simulink model "matlab_smith_opc_opre"  (R2018b)
settings: Solver=VariableStepAuto  StartTime=0.0  StopTime=40  RelTol=1e-3
undefined symbols (not defined in the file or in its folder): AI1, AO1, Dev1
libraries: opclib x3, simulink x1
settings Model: Creator=erange  LastModifiedBy=erange

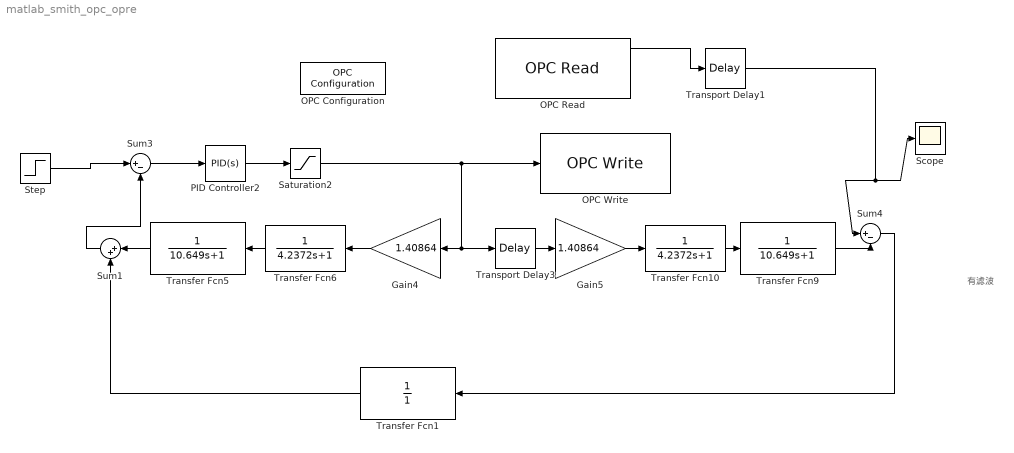
== system matlab_smith_opc_opre ==
  note: 有滤波
  Gain4 : Gain  Gain=1.40864
  Gain5 : Gain  Gain=1.40864
  OPC Configuration : opclib/OPC Configuration  opcServers=localhost/NI USB-6008.Server/10, localhost/Tank2.Server/10  errMissingItems=Error  errReadWrite=Warn  errShutdown=Error  errRTViolation=Warn  rtEnable=on  speedup=1  showLatency=off  beingUsed=on
      settings: SourceProductName=OPC Toolbox  SourceProductBaseCode=OT
  OPC Read : opclib/OPC Read  serverHost=localhost  serverID=NI USB-6008.Server  itemIDs=Dev1/AI1  readMode=Synchronous (cache)  dataType=double  updateRate=0.01  showQual=on  showTS=on  tsMode=Seconds since start
      settings: SourceProductName=OPC Toolbox  SourceProductBaseCode=OT
  OPC Write : opclib/OPC Write  serverHost=localhost  serverID=NI USB-6008.Server  itemIDs=Dev1/AO1  writeMode=Synchronous  updateRate=0.01
      settings: SourceProductName=OPC Toolbox  SourceProductBaseCode=OT
  PID Controller2 : simulink/Continuous/PID Controller  Controller=PID  Form=Ideal  TimeDomain=Continuous-time  SampleTime=0.1  IntegratorMethod=Forward Euler  FilterMethod=Forward Euler  ControllerParametersSource=internal  P=5  I=0.1  D=1.5  UseFilter=on  N=10000  TunerSelectOption=Transfer Function Based (PID Tuner App)  InitialConditionSource=internal  InitialConditionForIntegrator=0  InitialConditionForFilter=0  DifferentiatorICPrevScaledInput=0  ExternalReset=none  TrackingMode=off  Kt=1  LimitOutput=off  UpperSaturationLimit=inf  LowerSaturationLimit=-inf  LinearizeAsGain=on  AntiWindupMode=none  Kb=1  POutMin=[]  POutMax=[]  IOutMin=[]  IOutMax=[]  DOutMin=[]  DOutMax=[]  NOutMin=[]  NOutMax=[]  SumOutMin=[]  SumOutMax=[]  SaturationOutMin=[]  SaturationOutMax=[]  PParamMin=[]  PParamMax=[]  IParamMin=[]  IParamMax=[]  DParamMin=[]  DParamMax=[]  NParamMin=[]  NParamMax=[]  KbParamMin=[]  KbParamMax=[]  KtParamMin=[]  KtParamMax=[]  KbOutMin=[]  KbOutMax=[]  KtOutMin=[]  KtOutMax=[]  IntegratorOutMin=[]  IntegratorOutMax=[]  FilterOutMin=[]  FilterOutMax=[]  SumI1OutMin=[]  SumI1OutMax=[]  SumI2OutMin=[]  SumI2OutMax=[]  SumI3OutMin=[]  SumI3OutMax=[]  SumI4OutMin=[]  SumI4OutMax=[]  SumDOutMin=[]  SumDOutMax=[]  DifferentiatorOutMin=[]  DifferentiatorOutMax=[]  FilterDiffOutCoefMin=[]  FilterDiffOutCoefMax=[]  ReciprocalOutMin=[]  ReciprocalOutMax=[]  SumDenOutMin=[]  SumDenOutMax=[]  SumNumOutMin=[]  SumNumOutMax=[]  DivideOutMin=[]  DivideOutMax=[]  IntegratorContinuousStateAttributes=''  IntegratorStateMustResolveToSignalObject=off  IntegratorRTWStateStorageClass=Auto  FilterContinuousStateAttributes=''  FilterStateMustResolveToSignalObject=off  FilterRTWStateStorageClass=Auto  ParallelPVariant=Passthrough  IdealPVariant=InternalParameters  IVariant=InternalParameters  DVariant=InternalParameters  IntegratorVariant=Continuous  SatVariant=Disabled  AWVariant=Passthrough  PCopyVariant=Disabled  TRVariant=Disabled  FdbkBlocksVariant=Forward  IdealPFdbkVariant=Disabled  SatFdbkVariant=Disabled  DerivativeFilterVariant=ContFilter  NVariant=InternalParameters  NCopyVariant=Disabled  FilterICVariant=InternalICsFilter  IntegratorICVariant=InternalICs  ExternalResetVariant=Disabled  TRSumVariant=Passthrough  SumFdbkVariant=Disabled  SumVariant=Sum_PID
  Saturation2 : Saturate  UpperLimit=5  LowerLimit=0
  Scope : Scope
  Step : Step  Time=0  SampleTime=0
  Sum1 : Sum  Inputs=|++
  Sum3 : Sum  Inputs=|+-
  Sum4 : Sum  Inputs=|+-
  Transfer Fcn1 : TransferFcn  Denominator=[ 1]
  Transfer Fcn10 : TransferFcn  Denominator=[4.2372 1]
  Transfer Fcn5 : TransferFcn  Denominator=[10.649 1]
  Transfer Fcn6 : TransferFcn  Denominator=[4.2372 1]
  Transfer Fcn9 : TransferFcn  Denominator=[10.649 1]
  Transport Delay1 : TransportDelay  DelayTime=3
  Transport Delay3 : TransportDelay  DelayTime=3
  wires:
  Gain5/1 -> Transfer Fcn10/1
  Transfer Fcn9/1 -> Sum4/2
  Gain4/1 -> Transfer Fcn6/1
  Transfer Fcn10/1 -> Transfer Fcn9/1
  Transport Delay3/1 -> Gain5/1
  Transfer Fcn6/1 -> Transfer Fcn5/1
  Step/1 -> Sum3/1
  Saturation2/1 -> OPC Write/1, Gain4/1, Transport Delay3/1
  OPC Read/1 -> Transport Delay1/1
  Transport Delay1/1 -> Sum4/1, Scope/1
  PID Controller2/1 -> Saturation2/1
  Sum3/1 -> PID Controller2/1
  Transfer Fcn5/1 -> Sum1/1
  Sum1/1 -> Sum3/2
  Sum4/1 -> Transfer Fcn1/1
  Transfer Fcn1/1 -> Sum1/2
